simulink model "test_direct"  (R2024a)
settings: Solver=VariableStepAuto  StartTime=0.0  StopTime=40  RelTol=1e-3
libraries: neural x733, simulink x4
(part 24 of 35)

== system test_direct/Function Fitting Neural Network4/Layer 4/Delays 1 ==
  "p{4}" : Inport  PortDimensions=20
      mask Display: e = 0.06;c1 = [120 230 180]/255;c2 = ([120 230 180]+0)/(256+128);c3 = ([120 230 180]+128)/(256+128);patch([0 1 1 0],[0 0 1 1],c1);patch([0 1 1 1-e 1-e 0+e],[0 0 1 1-e 0+e 0+e],c2);patch([0 0 1 1-e 0+e 0+e],[0 1 1 1-e 1-e 0+e],c3);plot([0 1 1 0 0],[0 0 1 1 0]);
  mux : Mux  Inputs=1
      mask Display: e = 0.06;c1 = [120 150 230]/255;c2 = ([120 150 230]+0)/383;c3 = ([120 150 230]+128)/383;patch([0 1 1 0],[0 0 1 1],c1);patch([0 1 1 1-e 1-e 0+e],[0 0 1 1-e 0+e 0+e],c2);patch([0 0 1 1-e 0+e 0+e],[0 1 1 1-e 1-e 0+e],c3);plot([0 1 1 0 0],[0 0 1 1 0]);disp('Mux')
  "pd{4,3}" : Outport
      mask Display: e = 0.06;c1 = [120 230 180]/255;c2 = ([120 230 180]+0)/(256+128);c3 = ([120 230 180]+128)/(256+128);patch([0 1 1 0],[0 0 1 1],c1);patch([0 1 1 1-e 1-e 0+e],[0 0 1 1-e 0+e 0+e],c2);patch([0 0 1 1-e 0+e 0+e],[0 1 1 1-e 1-e 0+e],c3);plot([0 1 1 0 0],[0 0 1 1 0]);
  wires:
  "p{4}"/1 -> mux/1
  mux/1 -> "pd{4,3}"/1

== system test_direct/Function Fitting Neural Network4/Layer 4/LW{4,3} ==
  "ad{4,3}" : Inport  PortDimensions=20
      mask Display: e = 0.06;c1 = [120 230 180]/255;c2 = ([120 230 180]+0)/(256+128);c3 = ([120 230 180]+128)/(256+128);patch([0 1 1 0],[0 0 1 1],c1);patch([0 1 1 1-e 1-e 0+e],[0 0 1 1-e 0+e 0+e],c2);patch([0 0 1 1-e 0+e 0+e],[0 1 1 1-e 1-e 0+e],c3);plot([0 1 1 0 0],[0 0 1 1 0]);
  "IW{4,3}(1,:)'" : Constant  Value=[-0.0182808475685428926948983274769489071331918239593505859375;0.0804580234912133374081122383358888328075408935546875;-0.2073100011052473601314005691165220923721790313720703125;-0.56877624107405078124344299794756807386875152587890625;-0.37106551095573958587436891320976428687572479248046875;0.2453467469113256027579694773521623574197292327880859375;-0.1097157740776300016705135931260883808135986328125;0.293030747380307599048165911881369538605213165283203125;0.4286556952932023545344009107793681323528289794921875;-0.2927619933728118351012881248607300221920013427734375;-0.330831802187190826547436017790460027754306793212890625;-0.01300416253790542993329371057598109473474323749542236328125;-0.220024597925029985479028482586727477610111236572265625;0.28856741284184350693209353266865946352481842041015625;0.1738140495019694087286410422166227363049983978271484375;0.57653717402246307255353485743398778140544891357421875;-0.08144393527626341000580367790462332777678966522216796875;0.62386015914583803354531710283481515944004058837890625;0.23299635893419512466806509110028855502605438232421875;0.462827846568813539018805158775649033486843109130859375]
      mask Display: e = 0.06;c1 = [120 150 230]/255;c2 = ([120 150 230]+0)/383;c3 = ([120 150 230]+128)/383;patch([0 1 1 0],[0 0 1 1],c1);patch([0 1 1 1-e 1-e 0+e],[0 0 1 1-e 0+e 0+e],c2);patch([0 0 1 1-e 0+e 0+e],[0 1 1 1-e 1-e 0+e],c3);plot([0 1 1 0 0],[0 0 1 1 0]);disp('weights');
  "IW{4,3}(10,:)'" : Constant  Value=[-0.5867021051616487792301768422476015985012054443359375;-0.40646884911088843050919194865855388343334197998046875;0.1384930279966194444085658687981776893138885498046875;0.60431005202610743598512499374919570982456207275390625;0.231549088394502333709823460594634525477886199951171875;-0.278578383513912342106522146423230879008769989013671875;-0.2401723445859841599148154500653618015348911285400390625;-0.278682695857914330961335735992179252207279205322265625;0.389949189397055973049788235584856010973453521728515625;-0.378849241372464284882681795352254994213581085205078125;-0.50446895043893802412782179089845158159732818603515625;-0.04123499520558514264134686300167231820523738861083984375;-0.412512646032147267671774670816375873982906341552734375;0.0298074784018579376498880861845464096404612064361572265625;-0.6030020171920196236925448829424567520618438720703125;-0.0918971849790183037409718735943897627294063568115234375;-0.1048877360115925416739202091775950975716114044189453125;0.426138672134914464617594376250053755939006805419921875;-0.028373006982034938705528048785708961077034473419189453125;-0.10103546567123274091404283581141498871147632598876953125]
      mask Display: e = 0.06;c1 = [120 150 230]/255;c2 = ([120 150 230]+0)/383;c3 = ([120 150 230]+128)/383;patch([0 1 1 0],[0 0 1 1],c1);patch([0 1 1 1-e 1-e 0+e],[0 0 1 1-e 0+e 0+e],c2);patch([0 0 1 1-e 0+e 0+e],[0 1 1 1-e 1-e 0+e],c3);plot([0 1 1 0 0],[0 0 1 1 0]);disp('weights');
  "IW{4,3}(2,:)'" : Constant  Value=[0.04766233737430193573292314113132306374609470367431640625;0.472662950403235637697463289441657252609729766845703125;0.393481975518174265094017982846708036959171295166015625;-0.4054200644776970730021048439084552228450775146484375;0.64596436275341506672020841506309807300567626953125;0.34833116550052078963517487864010035991668701171875;0.0158927016381227755037475191102203098125755786895751953125;0.1432191124397620696218069724636734463274478912353515625;-0.1525863659129366445288411568981246091425418853759765625;-0.08213514792309771495038006605682312510907649993896484375;-0.05352653335257491484799885483880643732845783233642578125;-0.2237879229032577743652154822484590113162994384765625;-0.251639048104404128292088671514648012816905975341796875;0.374060271638200159127762844946119002997875213623046875;-0.13843849114586415094407811920973472297191619873046875;-0.00157935386633405584581868463800446988898329436779022216796875;0.08123459901137251859548626953255734406411647796630859375;-0.60194027599860344679427726077847182750701904296875;-0.2419573839009540316968838169486843980848789215087890625;0.4202479369474840797948900217306800186634063720703125]
      mask Display: e = 0.06;c1 = [120 150 230]/255;c2 = ([120 150 230]+0)/383;c3 = ([120 150 230]+128)/383;patch([0 1 1 0],[0 0 1 1],c1);patch([0 1 1 1-e 1-e 0+e],[0 0 1 1-e 0+e 0+e],c2);patch([0 0 1 1-e 0+e 0+e],[0 1 1 1-e 1-e 0+e],c3);plot([0 1 1 0 0],[0 0 1 1 0]);disp('weights');
  "IW{4,3}(3,:)'" : Constant  Value=[0.64653136532270083502993429647176526486873626708984375;-0.17598643231509558670921933298814110457897186279296875;-0.3306166204372065209327047341503202915191650390625;0.5500686330664434908754856223822571337223052978515625;-0.258915156366846421764904562223819084465503692626953125;-0.2135157354375183669237259209694457240402698516845703125;0.0280209258454371910873614837100831209681928157806396484375;0.023128965179387513118047792204379220493137836456298828125;0.300633725443321286885378640363342128694057464599609375;0.34519443371440450274434397215372882783412933349609375;-0.307061664525679400838953370111994445323944091796875;0.0201426192713053155147751027698177495039999485015869140625;0.1928095450190112358779259693619678728282451629638671875;-0.2828180192111175994540417377720586955547332763671875;0.67880942307011460368215693961246870458126068115234375;-0.18199528762274497228901282142032869160175323486328125;0.15160314165136490327512319709057919681072235107421875;0.48788420536031595897696888641803525388240814208984375;0.1995805530883998091251640971677261404693126678466796875;-0.39812724429761658928583756278385408222675323486328125]
      mask Display: e = 0.06;c1 = [120 150 230]/255;c2 = ([120 150 230]+0)/383;c3 = ([120 150 230]+128)/383;patch([0 1 1 0],[0 0 1 1],c1);patch([0 1 1 1-e 1-e 0+e],[0 0 1 1-e 0+e 0+e],c2);patch([0 0 1 1-e 0+e 0+e],[0 1 1 1-e 1-e 0+e],c3);plot([0 1 1 0 0],[0 0 1 1 0]);disp('weights');
  "IW{4,3}(4,:)'" : Constant  Value=[0.46897639649297795383375841993256472051143646240234375;0.1353316784521863269663555229271878488361835479736328125;-0.4090318643737698156570559149258770048618316650390625;-0.10034667176648993935916820419151918031275272369384765625;0.15356197843960306403943150144186802208423614501953125;-0.74982192036332262485842647947720251977443695068359375;0.736163475218127860699723896686919033527374267578125;-0.388099606476475178507001828620559535920619964599609375;0.1284378189965413030737551025595166720449924468994140625;-0.35342224141770184342448146708193235099315643310546875;0.33768468281888275317470515801687724888324737548828125;-0.33768459631601943637946305898367427289485931396484375;0.339246448835974323543496211641468107700347900390625;-0.182148817954333519519849460266414098441600799560546875;-0.45675022943742826786461819210671819746494293212890625;-0.1308331396638943433519131076536723412573337554931640625;0.007235920518857773438281544287065116805024445056915283203125;-0.2181989741993194120706078820148832164704799652099609375;0.697710740419517083665823520277626812458038330078125;0.03270757109621826030920743733076960779726505279541015625]
      mask Display: e = 0.06;c1 = [120 150 230]/255;c2 = ([120 150 230]+0)/383;c3 = ([120 150 230]+128)/383;patch([0 1 1 0],[0 0 1 1],c1);patch([0 1 1 1-e 1-e 0+e],[0 0 1 1-e 0+e 0+e],c2);patch([0 0 1 1-e 0+e 0+e],[0 1 1 1-e 1-e 0+e],c3);plot([0 1 1 0 0],[0 0 1 1 0]);disp('weights');
  "IW{4,3}(5,:)'" : Constant  Value=[0.254012415241254452258345963855390436947345733642578125;-0.278201611801674075774570837893406860530376434326171875;-0.130987915740999272262712338488199748098850250244140625;0.65659498971948615508864577350323088467121124267578125;-0.37010577209780526342086659496999345719814300537109375;-0.364239904557088711722911966717219911515712738037109375;-0.346218175332081823381003005124512128531932830810546875;-0.131514115645591733727570726841804571449756622314453125;-0.16293218459890457250338613448548130691051483154296875;-0.07690950801719813323398255988649907521903514862060546875;-0.04995568746558680384151074349574628286063671112060546875;-0.297894174787131815751450858442694880068302154541015625;-0.208190351516119920294300982277491129934787750244140625;-0.13629072817438714348980965951341204345226287841796875;-0.384110184134717147497184441817807964980602264404296875;-0.43900730118536801516171408366062678396701812744140625;0.0692901289663383213035530161505448631942272186279296875;0.27697027123827278050072209225618280470371246337890625;0.0208057391676239288036409647020263946615159511566162109375;0.6856311827603163155941956574679352343082427978515625]
      mask Display: e = 0.06;c1 = [120 150 230]/255;c2 = ([120 150 230]+0)/383;c3 = ([120 150 230]+128)/383;patch([0 1 1 0],[0 0 1 1],c1);patch([0 1 1 1-e 1-e 0+e],[0 0 1 1-e 0+e 0+e],c2);patch([0 0 1 1-e 0+e 0+e],[0 1 1 1-e 1-e 0+e],c3);plot([0 1 1 0 0],[0 0 1 1 0]);disp('weights');
  "IW{4,3}(6,:)'" : Constant  Value=[0.06383515321962386634968567022951901890337467193603515625;-0.348969499010585881837442912001279182732105255126953125;-0.67269644646642923202506381130660884082317352294921875;0.44685601061213520157622269834973849356174468994140625;-0.358281232233862712011074336260207928717136383056640625;0.07916658582745154937310161358254845254123210906982421875;0.30505773608176711686468252082704566419124603271484375;0.617951579143801499327537385397590696811676025390625;-0.25294218554518221875326844383380375802516937255859375;-0.3977997598759459574324637287645600736141204833984375;0.058739564042513479902307693691909662447869777679443359375;0.1494537664697459522500366801978088915348052978515625;0.60851330942889114705707243047072552144527435302734375;-0.055559362022579848738867980273425928317010402679443359375;-0.62443423379172180442964190660859458148479461669921875;-0.2268644620133335454426060096011497080326080322265625;-0.57816378248105604331641416138154454529285430908203125;0.39207408987547409662255404327879659831523895263671875;-0.074342103653326108148036155398585833609104156494140625;0.285697237530900871593786405355785973370075225830078125]
      mask Display: e = 0.06;c1 = [120 150 230]/255;c2 = ([120 150 230]+0)/383;c3 = ([120 150 230]+128)/383;patch([0 1 1 0],[0 0 1 1],c1);patch([0 1 1 1-e 1-e 0+e],[0 0 1 1-e 0+e 0+e],c2);patch([0 0 1 1-e 0+e 0+e],[0 1 1 1-e 1-e 0+e],c3);plot([0 1 1 0 0],[0 0 1 1 0]);disp('weights');
  "IW{4,3}(7,:)'" : Constant  Value=[0.1735578250848583692356186247707228176295757293701171875;-0.1443796965013408317712872985794092528522014617919921875;-0.00192713703805364963174417969327123500988818705081939697265625;-0.050944766962450170610932076442622928880155086517333984375;-0.56313960947635821607804018640308640897274017333984375;0.406795735506861155794666728979791514575481414794921875;-0.43477191912486556901740186731331050395965576171875;-0.0183635163924778209432187026095562032423913478851318359375;-0.16499808196158738393677367639611475169658660888671875;0.1554097258561016603461979457279085181653499603271484375;-0.45712271023931894120551078231073915958404541015625;-0.31639810290967407269135946989990770816802978515625;0.283675985048455980841453083485248498618602752685546875;-0.434852696669257132722208325503743253648281097412109375;0.184268928265691245282908994340687058866024017333984375;0.487799544058790834899497212973074056208133697509765625;-0.1646897501250245976489594568192842416465282440185546875;0.55969685707381255923564822296611964702606201171875;-0.40425367209081686237226449520676396787166595458984375;0.259423740372571154377823177128448151051998138427734375]
      mask Display: e = 0.06;c1 = [120 150 230]/255;c2 = ([120 150 230]+0)/383;c3 = ([120 150 230]+128)/383;patch([0 1 1 0],[0 0 1 1],c1);patch([0 1 1 1-e 1-e 0+e],[0 0 1 1-e 0+e 0+e],c2);patch([0 0 1 1-e 0+e 0+e],[0 1 1 1-e 1-e 0+e],c3);plot([0 1 1 0 0],[0 0 1 1 0]);disp('weights');
  "IW{4,3}(8,:)'" : Constant  Value=[-0.044604630833756091223829542968815076164901256561279296875;0.1653273492054885551727494430451770313084125518798828125;0.35228947713259184393308487415197305381298065185546875;0.388185803066177392839364301835303194820880889892578125;0.59881679713870406001063884104951284825801849365234375;-0.07736001152979880834958947843915666453540325164794921875;-0.5271011175306501428394767572171986103057861328125;-0.09774032952107626626148118020864785648882389068603515625;0.18675638954029449845251065198681317269802093505859375;-0.478571423377917526398306335977395065128803253173828125;0.34027059434836159912407538286061026155948638916015625;0.057705036219698628563445907957429881207644939422607421875;-0.214782881199087782864154405615408904850482940673828125;-0.26706306507587018739258155619609169661998748779296875;-0.54002602442711433727851044750423170626163482666015625;0.58528571806826767964793134524370543658733367919921875;0.030194751746646243673044551769635290838778018951416015625;-0.4346282259921803170499288171413354575634002685546875;0.40357189348227062719587365791085176169872283935546875;0.193904249336287748395335484019597060978412628173828125]
      mask Display: e = 0.06;c1 = [120 150 230]/255;c2 = ([120 150 230]+0)/383;c3 = ([120 150 230]+128)/383;patch([0 1 1 0],[0 0 1 1],c1);patch([0 1 1 1-e 1-e 0+e],[0 0 1 1-e 0+e 0+e],c2);patch([0 0 1 1-e 0+e 0+e],[0 1 1 1-e 1-e 0+e],c3);plot([0 1 1 0 0],[0 0 1 1 0]);disp('weights');
  "IW{4,3}(9,:)'" : Constant  Value=[-0.262696724536377546055376797085045836865901947021484375;-0.495272708083491608466175648572971113026142120361328125;-0.3543852059837149237608855401049368083477020263671875;-0.221393523730061769771992885580402798950672149658203125;-0.038436478394411034698041618185015977360308170318603515625;-0.318611608590077199920642669894732534885406494140625;-0.07339652443837078876764934420862118713557720184326171875;1.061095964250348355761843777145259082317352294921875;-0.4127361165109009188967092995881102979183197021484375;-0.025399426654827285398940972527270787395536899566650390625;-0.5236953508005728341601070496835745871067047119140625;-0.335822568857687187016125562877277843654155731201171875;0.350185935701288586496815469217835925519466400146484375;-0.195141267318745648129407754822750575840473175048828125;0.9131446131154741241431338494294323027133941650390625;-0.4326775227891754838083215872757136821746826171875;-0.63697775880777218748818313542869873344898223876953125;0.55100216042612715217074992324342019855976104736328125;-0.09919080628567943092033232233006856404244899749755859375;0.134968530413840992476792735033086501061916351318359375]
      mask Display: e = 0.06;c1 = [120 150 230]/255;c2 = ([120 150 230]+0)/383;c3 = ([120 150 230]+128)/383;patch([0 1 1 0],[0 0 1 1],c1);patch([0 1 1 1-e 1-e 0+e],[0 0 1 1-e 0+e 0+e],c2);patch([0 0 1 1-e 0+e 0+e],[0 1 1 1-e 1-e 0+e],c3);plot([0 1 1 0 0],[0 0 1 1 0]);disp('weights');
  Mux : Mux  Inputs=10
      mask Display: e = 0.06;c1 = [120 150 230]/255;c2 = ([120 150 230]+0)/383;c3 = ([120 150 230]+128)/383;patch([0 1 1 0],[0 0 1 1],c1);patch([0 1 1 1-e 1-e 0+e],[0 0 1 1-e 0+e 0+e],c2);patch([0 0 1 1-e 0+e 0+e],[0 1 1 1-e 1-e 0+e],c3);plot([0 1 1 0 0],[0 0 1 1 0]);disp('Mux');
  dotprod{1..10} (10 alike) : neural/Weight Functions/dotprod
  "lz{4,3}" : Outport
      mask Display: e = 0.06;c1 = [120 230 180]/255;c2 = ([120 230 180]+0)/(256+128);c3 = ([120 230 180]+128)/(256+128);patch([0 1 1 0],[0 0 1 1],c1);patch([0 1 1 1-e 1-e 0+e],[0 0 1 1-e 0+e 0+e],c2);patch([0 0 1 1-e 0+e 0+e],[0 1 1 1-e 1-e 0+e],c3);plot([0 1 1 0 0],[0 0 1 1 0]);
  wires:
  "IW{4,3}(1,:)'"/1 -> dotprod1/1
  "ad{4,3}"/1 -> dotprod1/2, dotprod2/2, dotprod3/2, dotprod4/2, dotprod5/2, dotprod6/2, dotprod7/2, dotprod8/2, dotprod9/2, dotprod10/2
  dotprod1/1 -> Mux/1
  "IW{4,3}(2,:)'"/1 -> dotprod2/1
  dotprod2/1 -> Mux/2
  "IW{4,3}(3,:)'"/1 -> dotprod3/1
  dotprod3/1 -> Mux/3
  "IW{4,3}(4,:)'"/1 -> dotprod4/1
  dotprod4/1 -> Mux/4
  "IW{4,3}(5,:)'"/1 -> dotprod5/1
  dotprod5/1 -> Mux/5
  "IW{4,3}(6,:)'"/1 -> dotprod6/1
  dotprod6/1 -> Mux/6
  "IW{4,3}(7,:)'"/1 -> dotprod7/1
  dotprod7/1 -> Mux/7
  "IW{4,3}(8,:)'"/1 -> dotprod8/1
  dotprod8/1 -> Mux/8
  "IW{4,3}(9,:)'"/1 -> dotprod9/1
  dotprod9/1 -> Mux/9
  "IW{4,3}(10,:)'"/1 -> dotprod10/1
  dotprod10/1 -> Mux/10
  Mux/1 -> "lz{4,3}"/1

== system test_direct/Function Fitting Neural Network4/Layer 5/Delays 1 ==
  "p{5}" : Inport  PortDimensions=10
      mask Display: e = 0.06;c1 = [120 230 180]/255;c2 = ([120 230 180]+0)/(256+128);c3 = ([120 230 180]+128)/(256+128);patch([0 1 1 0],[0 0 1 1],c1);patch([0 1 1 1-e 1-e 0+e],[0 0 1 1-e 0+e 0+e],c2);patch([0 0 1 1-e 0+e 0+e],[0 1 1 1-e 1-e 0+e],c3);plot([0 1 1 0 0],[0 0 1 1 0]);
  mux : Mux  Inputs=1
      mask Display: e = 0.06;c1 = [120 150 230]/255;c2 = ([120 150 230]+0)/383;c3 = ([120 150 230]+128)/383;patch([0 1 1 0],[0 0 1 1],c1);patch([0 1 1 1-e 1-e 0+e],[0 0 1 1-e 0+e 0+e],c2);patch([0 0 1 1-e 0+e 0+e],[0 1 1 1-e 1-e 0+e],c3);plot([0 1 1 0 0],[0 0 1 1 0]);disp('Mux')
  "pd{5,4}" : Outport
      mask Display: e = 0.06;c1 = [120 230 180]/255;c2 = ([120 230 180]+0)/(256+128);c3 = ([120 230 180]+128)/(256+128);patch([0 1 1 0],[0 0 1 1],c1);patch([0 1 1 1-e 1-e 0+e],[0 0 1 1-e 0+e 0+e],c2);patch([0 0 1 1-e 0+e 0+e],[0 1 1 1-e 1-e 0+e],c3);plot([0 1 1 0 0],[0 0 1 1 0]);
  wires:
  "p{5}"/1 -> mux/1
  mux/1 -> "pd{5,4}"/1

== system test_direct/Function Fitting Neural Network4/Layer 5/LW{5,4} ==
  "ad{5,4}" : Inport  PortDimensions=10
      mask Display: e = 0.06;c1 = [120 230 180]/255;c2 = ([120 230 180]+0)/(256+128);c3 = ([120 230 180]+128)/(256+128);patch([0 1 1 0],[0 0 1 1],c1);patch([0 1 1 1-e 1-e 0+e],[0 0 1 1-e 0+e 0+e],c2);patch([0 0 1 1-e 0+e 0+e],[0 1 1 1-e 1-e 0+e],c3);plot([0 1 1 0 0],[0 0 1 1 0]);
  "IW{5,4}(1,:)'" : Constant  Value=[-0.609586613853234648985335297766141593456268310546875;-0.991992343621268535258650445030070841312408447265625;0.55645920623334166332796257847803644835948944091796875;-0.2756548382209949021870443175430409610271453857421875;0.79182679604217509616859160814783535897731781005859375;0.5409353217326822171884259660146199166774749755859375;0.8560146531317720519638214682345278561115264892578125;0.369094621261524424848943226606934331357479095458984375;1.144450010398711636838697813800536096096038818359375;0.82688754328264491011424297539633698761463165283203125]
      mask Display: e = 0.06;c1 = [120 150 230]/255;c2 = ([120 150 230]+0)/383;c3 = ([120 150 230]+128)/383;patch([0 1 1 0],[0 0 1 1],c1);patch([0 1 1 1-e 1-e 0+e],[0 0 1 1-e 0+e 0+e],c2);patch([0 0 1 1-e 0+e 0+e],[0 1 1 1-e 1-e 0+e],c3);plot([0 1 1 0 0],[0 0 1 1 0]);disp('weights');
  "IW{5,4}(2,:)'" : Constant  Value=[-0.2491134788551136736156621509508113376796245574951171875;-0.348638402621329834829566607368178665637969970703125;-0.58928454736647262190984974949969910085201263427734375;1.1057017527083596863946013399981893599033355712890625;0.69839147102565746205726782136480323970317840576171875;-0.78717405206411239504404875333420932292938232421875;0.1763952297557981607756261155373067595064640045166015625;-0.0641150518456101436992611297682742588222026824951171875;-0.9062580556750947646804661417263559997081756591796875;-1.0565207862803387417471867593121714890003204345703125]
      mask Display: e = 0.06;c1 = [120 150 230]/255;c2 = ([120 150 230]+0)/383;c3 = ([120 150 230]+128)/383;patch([0 1 1 0],[0 0 1 1],c1);patch([0 1 1 1-e 1-e 0+e],[0 0 1 1-e 0+e 0+e],c2);patch([0 0 1 1-e 0+e 0+e],[0 1 1 1-e 1-e 0+e],c3);plot([0 1 1 0 0],[0 0 1 1 0]);disp('weights');
  Mux : Mux  Inputs=2
      mask Display: e = 0.06;c1 = [120 150 230]/255;c2 = ([120 150 230]+0)/383;c3 = ([120 150 230]+128)/383;patch([0 1 1 0],[0 0 1 1],c1);patch([0 1 1 1-e 1-e 0+e],[0 0 1 1-e 0+e 0+e],c2);patch([0 0 1 1-e 0+e 0+e],[0 1 1 1-e 1-e 0+e],c3);plot([0 1 1 0 0],[0 0 1 1 0]);disp('Mux');
  dotprod1 : neural/Weight Functions/dotprod
  dotprod2 : neural/Weight Functions/dotprod
  "lz{5,4}" : Outport
      mask Display: e = 0.06;c1 = [120 230 180]/255;c2 = ([120 230 180]+0)/(256+128);c3 = ([120 230 180]+128)/(256+128);patch([0 1 1 0],[0 0 1 1],c1);patch([0 1 1 1-e 1-e 0+e],[0 0 1 1-e 0+e 0+e],c2);patch([0 0 1 1-e 0+e 0+e],[0 1 1 1-e 1-e 0+e],c3);plot([0 1 1 0 0],[0 0 1 1 0]);
  wires:
  "IW{5,4}(1,:)'"/1 -> dotprod1/1
  "ad{5,4}"/1 -> dotprod1/2, dotprod2/2
  dotprod1/1 -> Mux/1
  "IW{5,4}(2,:)'"/1 -> dotprod2/1
  dotprod2/1 -> Mux/2
  Mux/1 -> "lz{5,4}"/1

== system test_direct/Function Fitting Neural Network5/Layer 1/Delays 1 ==
  "p{1}" : Inport  PortDimensions=8
      mask Display: e = 0.06;c1 = [120 230 180]/255;c2 = ([120 230 180]+0)/(256+128);c3 = ([120 230 180]+128)/(256+128);patch([0 1 1 0],[0 0 1 1],c1);patch([0 1 1 1-e 1-e 0+e],[0 0 1 1-e 0+e 0+e],c2);patch([0 0 1 1-e 0+e 0+e],[0 1 1 1-e 1-e 0+e],c3);plot([0 1 1 0 0],[0 0 1 1 0]);
  mux : Mux  Inputs=1
      mask Display: e = 0.06;c1 = [120 150 230]/255;c2 = ([120 150 230]+0)/383;c3 = ([120 150 230]+128)/383;patch([0 1 1 0],[0 0 1 1],c1);patch([0 1 1 1-e 1-e 0+e],[0 0 1 1-e 0+e 0+e],c2);patch([0 0 1 1-e 0+e 0+e],[0 1 1 1-e 1-e 0+e],c3);plot([0 1 1 0 0],[0 0 1 1 0]);disp('Mux')
  "pd{1,1}" : Outport
      mask Display: e = 0.06;c1 = [120 230 180]/255;c2 = ([120 230 180]+0)/(256+128);c3 = ([120 230 180]+128)/(256+128);patch([0 1 1 0],[0 0 1 1],c1);patch([0 1 1 1-e 1-e 0+e],[0 0 1 1-e 0+e 0+e],c2);patch([0 0 1 1-e 0+e 0+e],[0 1 1 1-e 1-e 0+e],c3);plot([0 1 1 0 0],[0 0 1 1 0]);
  wires:
  "p{1}"/1 -> mux/1
  mux/1 -> "pd{1,1}"/1

== system test_direct/Function Fitting Neural Network5/Layer 1/IW{1,1} ==
  "pd{1,1}" : Inport  PortDimensions=8
      mask Display: e = 0.06;c1 = [120 230 180]/255;c2 = ([120 230 180]+0)/(256+128);c3 = ([120 230 180]+128)/(256+128);patch([0 1 1 0],[0 0 1 1],c1);patch([0 1 1 1-e 1-e 0+e],[0 0 1 1-e 0+e 0+e],c2);patch([0 0 1 1-e 0+e 0+e],[0 1 1 1-e 1-e 0+e],c3);plot([0 1 1 0 0],[0 0 1 1 0]);
  "IW{1,1}(1,:)'" : Constant  Value=[-0.24282240031374058286672834583441726863384246826171875;-0.265937760938790013209853668740834109485149383544921875;0.120517267596000288154556301378761418163776397705078125;-0.1509670298731921878054862418139236979186534881591796875;-0.83895200425768745589039099286310374736785888671875;-0.90347229810113471870636203675530850887298583984375;0.68495171502979490529838813017704524099826812744140625;0.956494783351313326846820928039960563182830810546875]
      mask Display: e = 0.06;c1 = [120 150 230]/255;c2 = ([120 150 230]+0)/383;c3 = ([120 150 230]+128)/383;patch([0 1 1 0],[0 0 1 1],c1);patch([0 1 1 1-e 1-e 0+e],[0 0 1 1-e 0+e 0+e],c2);patch([0 0 1 1-e 0+e 0+e],[0 1 1 1-e 1-e 0+e],c3);plot([0 1 1 0 0],[0 0 1 1 0]);disp('Weights');
  "IW{1,1}(10,:)'" : Constant  Value=[0.02780686991910841232567008773912675678730010986328125;0.0146068261959116096893041003568214364349842071533203125;-0.2385781861446483187449985052808187901973724365234375;0.1297828418770725911191021850754623301327228546142578125;0.5661070405517631964897873331210575997829437255859375;2.4081053896491244614708193694241344928741455078125;-0.6291887482895004435334840309224091470241546630859375;-0.3738127625013678567711394862271845340728759765625]
      mask Display: e = 0.06;c1 = [120 150 230]/255;c2 = ([120 150 230]+0)/383;c3 = ([120 150 230]+128)/383;patch([0 1 1 0],[0 0 1 1],c1);patch([0 1 1 1-e 1-e 0+e],[0 0 1 1-e 0+e 0+e],c2);patch([0 0 1 1-e 0+e 0+e],[0 1 1 1-e 1-e 0+e],c3);plot([0 1 1 0 0],[0 0 1 1 0]);disp('Weights');
  "IW{1,1}(11,:)'" : Constant  Value=[0.0015329316616055177306676693405051992158405482769012451171875;-0.004795595490663421937849175691326308879069983959197998046875;-0.2186967381351949679668678072630427777767181396484375;-0.04411631562895602931551053416114882566034793853759765625;1.0178167415469101531044771036249585449695587158203125;-0.355344103689434753778897402298753149807453155517578125;-0.9652366094281610298111218071426264941692352294921875;1.957180430553698169404697182471863925457000732421875]
      mask Display: e = 0.06;c1 = [120 150 230]/255;c2 = ([120 150 230]+0)/383;c3 = ([120 150 230]+128)/383;patch([0 1 1 0],[0 0 1 1],c1);patch([0 1 1 1-e 1-e 0+e],[0 0 1 1-e 0+e 0+e],c2);patch([0 0 1 1-e 0+e 0+e],[0 1 1 1-e 1-e 0+e],c3);plot([0 1 1 0 0],[0 0 1 1 0]);disp('Weights');
  "IW{1,1}(12,:)'" : Constant  Value=[0.033997681110883908039976830650630290620028972625732421875;0.037387204982984804935153277938297833316028118133544921875;1.2241007003313961742918536401703022420406341552734375;0.989772821617917575309775202185846865177154541015625;1.015743601330306500329925256664864718914031982421875;0.85100263802785980349341343753621913492679595947265625;-1.09811263426762995010221857228316366672515869140625;0.76300254608823314672605420128093101084232330322265625]
      mask Display: e = 0.06;c1 = [120 150 230]/255;c2 = ([120 150 230]+0)/383;c3 = ([120 150 230]+128)/383;patch([0 1 1 0],[0 0 1 1],c1);patch([0 1 1 1-e 1-e 0+e],[0 0 1 1-e 0+e 0+e],c2);patch([0 0 1 1-e 0+e 0+e],[0 1 1 1-e 1-e 0+e],c3);plot([0 1 1 0 0],[0 0 1 1 0]);disp('Weights');
  "IW{1,1}(13,:)'" : Constant  Value=[-0.00584867446382439197527514096464074100367724895477294921875;-0.014180135875496387154459654311722260899841785430908203125;0.048262697432363992067205771263616043142974376678466796875;-0.04770492383946049741449968450979213230311870574951171875;-0.420740831146248550620470041394582949578762054443359375;0.65870243261579342064493403086089529097080230712890625;0.6527847868744454107314822977059520781040191650390625;-0.2595271311505620293047513769124634563922882080078125]
      mask Display: e = 0.06;c1 = [120 150 230]/255;c2 = ([120 150 230]+0)/383;c3 = ([120 150 230]+128)/383;patch([0 1 1 0],[0 0 1 1],c1);patch([0 1 1 1-e 1-e 0+e],[0 0 1 1-e 0+e 0+e],c2);patch([0 0 1 1-e 0+e 0+e],[0 1 1 1-e 1-e 0+e],c3);plot([0 1 1 0 0],[0 0 1 1 0]);disp('Weights');
  "IW{1,1}(14,:)'" : Constant  Value=[0.3832677484937174750001531720045022666454315185546875;0.236375390594321832526958360176649875938892364501953125;-0.307434790104118338405214672093279659748077392578125;-0.75973655151750119074449685285799205303192138671875;0.6249548206558639407148803002201020717620849609375;0.330795354589032253311842168841394595801830291748046875;1.103439605613709684206469319178722798824310302734375;0.51173857903875286101680330830276943743228912353515625]
      mask Display: e = 0.06;c1 = [120 150 230]/255;c2 = ([120 150 230]+0)/383;c3 = ([120 150 230]+128)/383;patch([0 1 1 0],[0 0 1 1],c1);patch([0 1 1 1-e 1-e 0+e],[0 0 1 1-e 0+e 0+e],c2);patch([0 0 1 1-e 0+e 0+e],[0 1 1 1-e 1-e 0+e],c3);plot([0 1 1 0 0],[0 0 1 1 0]);disp('Weights');
  "IW{1,1}(15,:)'" : Constant  Value=[-0.1830343037830250707553858546816627494990825653076171875;-0.11318758575875147165401557458608294837176799774169921875;0.8364186150389627538714876209269277751445770263671875;0.108692940292483275488422123089549131691455841064453125;-0.8925071740038299505926033816649578511714935302734375;0.37947416924861177012218149684485979378223419189453125;-0.64906408913662427817570232946309261023998260498046875;-0.395045848186393377954317429612274281680583953857421875]
      mask Display: e = 0.06;c1 = [120 150 230]/255;c2 = ([120 150 230]+0)/383;c3 = ([120 150 230]+128)/383;patch([0 1 1 0],[0 0 1 1],c1);patch([0 1 1 1-e 1-e 0+e],[0 0 1 1-e 0+e 0+e],c2);patch([0 0 1 1-e 0+e 0+e],[0 1 1 1-e 1-e 0+e],c3);plot([0 1 1 0 0],[0 0 1 1 0]);disp('Weights');
  "IW{1,1}(16,:)'" : Constant  Value=[-0.01364560598087976965586687327913750777952373027801513671875;-0.04442535095315698623341660322694224305450916290283203125;-1.02925763778331447184655189630575478076934814453125;-0.791757846898343498054373412742279469966888427734375;0.404037544222803524096576666124747134745121002197265625;1.1093011870314255506997369593591429293155670166015625;-0.2280039202570558476423911997699178755283355712890625;-0.78285864379998482132094750340911559760570526123046875]
      mask Display: e = 0.06;c1 = [120 150 230]/255;c2 = ([120 150 230]+0)/383;c3 = ([120 150 230]+128)/383;patch([0 1 1 0],[0 0 1 1],c1);patch([0 1 1 1-e 1-e 0+e],[0 0 1 1-e 0+e 0+e],c2);patch([0 0 1 1-e 0+e 0+e],[0 1 1 1-e 1-e 0+e],c3);plot([0 1 1 0 0],[0 0 1 1 0]);disp('Weights');
  "IW{1,1}(17,:)'" : Constant  Value=[-0.2553234117613261133783453260548412799835205078125;-0.1392227370325401503148299298118217848241329193115234375;0.91924864981972020938627565556089393794536590576171875;0.6145246696287907095523905809386633336544036865234375;-0.95063315123071834289447679111617617309093475341796875;0.0742980094308140770476001080169226042926311492919921875;-0.447293047826839984537627969984896481037139892578125;-0.07736378923439117538674025809086742810904979705810546875]
      mask Display: e = 0.06;c1 = [120 150 230]/255;c2 = ([120 150 230]+0)/383;c3 = ([120 150 230]+128)/383;patch([0 1 1 0],[0 0 1 1],c1);patch([0 1 1 1-e 1-e 0+e],[0 0 1 1-e 0+e 0+e],c2);patch([0 0 1 1-e 0+e 0+e],[0 1 1 1-e 1-e 0+e],c3);plot([0 1 1 0 0],[0 0 1 1 0]);disp('Weights');
  "IW{1,1}(18,:)'" : Constant  Value=[-0.42587133665593823739214940360398031771183013916015625;-0.6138615427850846462121126023703254759311676025390625;-0.2327288350323049315182544205526937730610370635986328125;-0.2276120255623092225594206183814094401895999908447265625;-0.506769106523939694142200096393935382366180419921875;0.308581830945979185276684120253776200115680694580078125;-0.6815697384903725009053232497535645961761474609375;-0.1477754211640225079360533300132374279201030731201171875]
      mask Display: e = 0.06;c1 = [120 150 230]/255;c2 = ([120 150 230]+0)/383;c3 = ([120 150 230]+128)/383;patch([0 1 1 0],[0 0 1 1],c1);patch([0 1 1 1-e 1-e 0+e],[0 0 1 1-e 0+e 0+e],c2);patch([0 0 1 1-e 0+e 0+e],[0 1 1 1-e 1-e 0+e],c3);plot([0 1 1 0 0],[0 0 1 1 0]);disp('Weights');
  "IW{1,1}(19,:)'" : Constant  Value=[0.379732293415370403266706489375792443752288818359375;-0.1595555519094243035471691882776212878525257110595703125;0.950318483165697447390130037092603743076324462890625;-0.89054163698607868848711177633958868682384490966796875;-0.77398786886086490266478676858241669833660125732421875;0.355933090379061900510038185529992915689945220947265625;0.41853242967000114926889864364056847989559173583984375;0.72254742801642490857005896032205782830715179443359375]
      mask Display: e = 0.06;c1 = [120 150 230]/255;c2 = ([120 150 230]+0)/383;c3 = ([120 150 230]+128)/383;patch([0 1 1 0],[0 0 1 1],c1);patch([0 1 1 1-e 1-e 0+e],[0 0 1 1-e 0+e 0+e],c2);patch([0 0 1 1-e 0+e 0+e],[0 1 1 1-e 1-e 0+e],c3);plot([0 1 1 0 0],[0 0 1 1 0]);disp('Weights');
  "IW{1,1}(2,:)'" : Constant  Value=[0.503765398757633153792312441510148346424102783203125;0.34728427513297421835858358463156037032604217529296875;-1.096710226166195401020786448498256504535675048828125;0.462784035857158493332264015407417900860309600830078125;-0.89913794079431463845963889980339445173740386962890625;-0.1626930692858376270581999278874718584120273590087890625;0.369386693508937880014997290345490910112857818603515625;1.0995296511180006060470759621239267289638519287109375]
      mask Display: e = 0.06;c1 = [120 150 230]/255;c2 = ([120 150 230]+0)/383;c3 = ([120 150 230]+128)/383;patch([0 1 1 0],[0 0 1 1],c1);patch([0 1 1 1-e 1-e 0+e],[0 0 1 1-e 0+e 0+e],c2);patch([0 0 1 1-e 0+e 0+e],[0 1 1 1-e 1-e 0+e],c3);plot([0 1 1 0 0],[0 0 1 1 0]);disp('Weights');
  "IW{1,1}(20,:)'" : Constant  Value=[-0.463500722353860583613283097292878665030002593994140625;-0.81599737722350607072030470590107142925262451171875;-0.32719783735946383895765166016644798219203948974609375;-0.40053384670856784222081614643684588372707366943359375;0.63899774146409271669000418114592321217060089111328125;-0.64006294689625675697897122518043033778667449951171875;-0.44045233745919254442213741640443913638591766357421875;-0.08168367648872841557672330736750154756009578704833984375]
      mask Display: e = 0.06;c1 = [120 150 230]/255;c2 = ([120 150 230]+0)/383;c3 = ([120 150 230]+128)/383;patch([0 1 1 0],[0 0 1 1],c1);patch([0 1 1 1-e 1-e 0+e],[0 0 1 1-e 0+e 0+e],c2);patch([0 0 1 1-e 0+e 0+e],[0 1 1 1-e 1-e 0+e],c3);plot([0 1 1 0 0],[0 0 1 1 0]);disp('Weights');
  "IW{1,1}(3,:)'" : Constant  Value=[0.0723748364916112496558753264253027737140655517578125;0.06899037104716111701296910041492083109915256500244140625;0.0231040778098698072751115972778279683552682399749755859375;0.01373786016838408723106379483169803279452025890350341796875;-0.36868446239069119219067260928568430244922637939453125;0.7486580629124144348196523424121551215648651123046875;-0.2346237311682986825811525477547547779977321624755859375;-1.0772597850419514120545727564604021608829498291015625]
      mask Display: e = 0.06;c1 = [120 150 230]/255;c2 = ([120 150 230]+0)/383;c3 = ([120 150 230]+128)/383;patch([0 1 1 0],[0 0 1 1],c1);patch([0 1 1 1-e 1-e 0+e],[0 0 1 1-e 0+e 0+e],c2);patch([0 0 1 1-e 0+e 0+e],[0 1 1 1-e 1-e 0+e],c3);plot([0 1 1 0 0],[0 0 1 1 0]);disp('Weights');
  "IW{1,1}(4,:)'" : Constant  Value=[-0.01154571316516157623854876845825856435112655162811279296875;-0.015918434301198040869973482358545879833400249481201171875;-0.33500553416689882180179438364575617015361785888671875;-0.1741814446284809247966762768555781804025173187255859375;1.0290956808094076091464330602320842444896697998046875;-0.25840013824531415931318178991205058991909027099609375;-0.86294512365705833278894942850456573069095611572265625;1.9706795080646621887154879004810936748981475830078125]
      mask Display: e = 0.06;c1 = [120 150 230]/255;c2 = ([120 150 230]+0)/383;c3 = ([120 150 230]+128)/383;patch([0 1 1 0],[0 0 1 1],c1);patch([0 1 1 1-e 1-e 0+e],[0 0 1 1-e 0+e 0+e],c2);patch([0 0 1 1-e 0+e 0+e],[0 1 1 1-e 1-e 0+e],c3);plot([0 1 1 0 0],[0 0 1 1 0]);disp('Weights');
  "IW{1,1}(5,:)'" : Constant  Value=[-0.01049457889926454744189410206445245421491563320159912109375;-0.035729863245095937196449398243203177116811275482177734375;-0.430774484447114358598440730929723940789699554443359375;-0.0402661741306189480127386559615842998027801513671875;-0.176857648442543757827394301784806884825229644775390625;0.092448046676315509539989534459891729056835174560546875;0.155069558594852330291047337595955468714237213134765625;2.11663540805323346916111404425464570522308349609375]
      mask Display: e = 0.06;c1 = [120 150 230]/255;c2 = ([120 150 230]+0)/383;c3 = ([120 150 230]+128)/383;patch([0 1 1 0],[0 0 1 1],c1);patch([0 1 1 1-e 1-e 0+e],[0 0 1 1-e 0+e 0+e],c2);patch([0 0 1 1-e 0+e 0+e],[0 1 1 1-e 1-e 0+e],c3);plot([0 1 1 0 0],[0 0 1 1 0]);disp('Weights');
  "IW{1,1}(6,:)'" : Constant  Value=[-0.051120531659696322179797789431177079677581787109375;-0.1469645095613345830987128692868282087147235870361328125;-0.1943630337617625880586302855590474791824817657470703125;-0.0862961248053733254170793998127919621765613555908203125;0.2213018685352453884807033546167076565325260162353515625;-0.463147109011033009107194402531604282557964324951171875;-0.2054205721774859938477675314061343669891357421875;-1.9274833003906526318615988202509470283985137939453125]
      mask Display: e = 0.06;c1 = [120 150 230]/255;c2 = ([120 150 230]+0)/383;c3 = ([120 150 230]+128)/383;patch([0 1 1 0],[0 0 1 1],c1);patch([0 1 1 1-e 1-e 0+e],[0 0 1 1-e 0+e 0+e],c2);patch([0 0 1 1-e 0+e 0+e],[0 1 1 1-e 1-e 0+e],c3);plot([0 1 1 0 0],[0 0 1 1 0]);disp('Weights');
  "IW{1,1}(7,:)'" : Constant  Value=[-0.00350074955720112469814697675474235438741743564605712890625;-0.01146075157482118016261107840136901359073817729949951171875;-0.154440964692578008854439985952922143042087554931640625;-0.06737032278262101991916921406300389207899570465087890625;-1.3233228734849655783278876697295345366001129150390625;0.91760714123268216635409544323920272290706634521484375;1.3691568614437079620671511293039657175540924072265625;0.373878014397877489471966327982954680919647216796875]
      mask Display: e = 0.06;c1 = [120 150 230]/255;c2 = ([120 150 230]+0)/383;c3 = ([120 150 230]+128)/383;patch([0 1 1 0],[0 0 1 1],c1);patch([0 1 1 1-e 1-e 0+e],[0 0 1 1-e 0+e 0+e],c2);patch([0 0 1 1-e 0+e 0+e],[0 1 1 1-e 1-e 0+e],c3);plot([0 1 1 0 0],[0 0 1 1 0]);disp('Weights');
  "IW{1,1}(8,:)'" : Constant  Value=[-0.0240972952959477883239092221856481046415865421295166015625;-0.0118753658992399833971287392841986729763448238372802734375;-0.73527702222140745025313890437246300280094146728515625;-0.38907272860587360785444843713776208460330963134765625;1.020545316067873020671186168328858911991119384765625;-0.411154739334674612649678238085471093654632568359375;-0.95343221002979039457869703255710192024707794189453125;-0.1531734423163644276399963928270153701305389404296875]
      mask Display: e = 0.06;c1 = [120 150 230]/255;c2 = ([120 150 230]+0)/383;c3 = ([120 150 230]+128)/383;patch([0 1 1 0],[0 0 1 1],c1);patch([0 1 1 1-e 1-e 0+e],[0 0 1 1-e 0+e 0+e],c2);patch([0 0 1 1-e 0+e 0+e],[0 1 1 1-e 1-e 0+e],c3);plot([0 1 1 0 0],[0 0 1 1 0]);disp('Weights');
  "IW{1,1}(9,:)'" : Constant  Value=[0.0047450332710312383144302117443658062256872653961181640625;0.0092865309018203383295553265952548827044665813446044921875;-0.041284326840054286211767475833767093718051910400390625;0.0193521567803049132638903984116041101515293121337890625;-0.234218092953510759191004808599245734512805938720703125;-0.59102796727611262017632043352932669222354888916015625;0.52631472028489623138369779553613625466823577880859375;0.678027589694444099421843930031172931194305419921875]
      mask Display: e = 0.06;c1 = [120 150 230]/255;c2 = ([120 150 230]+0)/383;c3 = ([120 150 230]+128)/383;patch([0 1 1 0],[0 0 1 1],c1);patch([0 1 1 1-e 1-e 0+e],[0 0 1 1-e 0+e 0+e],c2);patch([0 0 1 1-e 0+e 0+e],[0 1 1 1-e 1-e 0+e],c3);plot([0 1 1 0 0],[0 0 1 1 0]);disp('Weights');
  Mux : Mux  Inputs=20
      mask Display: e = 0.06;c1 = [120 150 230]/255;c2 = ([120 150 230]+0)/383;c3 = ([120 150 230]+128)/383;patch([0 1 1 0],[0 0 1 1],c1);patch([0 1 1 1-e 1-e 0+e],[0 0 1 1-e 0+e 0+e],c2);patch([0 0 1 1-e 0+e 0+e],[0 1 1 1-e 1-e 0+e],c3);plot([0 1 1 0 0],[0 0 1 1 0]);disp('Mux');
  dotprod{1..20} (20 alike) : neural/Weight Functions/dotprod
  "iz{1,1}" : Outport
      mask Display: e = 0.06;c1 = [120 230 180]/255;c2 = ([120 230 180]+0)/(256+128);c3 = ([120 230 180]+128)/(256+128);patch([0 1 1 0],[0 0 1 1],c1);patch([0 1 1 1-e 1-e 0+e],[0 0 1 1-e 0+e 0+e],c2);patch([0 0 1 1-e 0+e 0+e],[0 1 1 1-e 1-e 0+e],c3);plot([0 1 1 0 0],[0 0 1 1 0]);
  wires:
  "IW{1,1}(1,:)'"/1 -> dotprod1/1
  "pd{1,1}"/1 -> dotprod1/2, dotprod2/2, dotprod3/2, dotprod4/2, dotprod5/2, dotprod6/2, dotprod7/2, dotprod8/2, dotprod9/2, dotprod10/2, dotprod11/2, dotprod12/2, dotprod13/2, dotprod14/2, dotprod15/2, dotprod16/2, dotprod17/2, dotprod18/2, dotprod19/2, dotprod20/2
  dotprod1/1 -> Mux/1
  "IW{1,1}(2,:)'"/1 -> dotprod2/1
  dotprod2/1 -> Mux/2
  "IW{1,1}(3,:)'"/1 -> dotprod3/1
  dotprod3/1 -> Mux/3
  "IW{1,1}(4,:)'"/1 -> dotprod4/1
  dotprod4/1 -> Mux/4
  "IW{1,1}(5,:)'"/1 -> dotprod5/1
  dotprod5/1 -> Mux/5
  "IW{1,1}(6,:)'"/1 -> dotprod6/1
  dotprod6/1 -> Mux/6
  "IW{1,1}(7,:)'"/1 -> dotprod7/1
  dotprod7/1 -> Mux/7
  "IW{1,1}(8,:)'"/1 -> dotprod8/1
  dotprod8/1 -> Mux/8
  "IW{1,1}(9,:)'"/1 -> dotprod9/1
  dotprod9/1 -> Mux/9
  "IW{1,1}(10,:)'"/1 -> dotprod10/1
  dotprod10/1 -> Mux/10
  "IW{1,1}(11,:)'"/1 -> dotprod11/1
  dotprod11/1 -> Mux/11
  "IW{1,1}(12,:)'"/1 -> dotprod12/1
  dotprod12/1 -> Mux/12
  "IW{1,1}(13,:)'"/1 -> dotprod13/1
  dotprod13/1 -> Mux/13
  "IW{1,1}(14,:)'"/1 -> dotprod14/1
  dotprod14/1 -> Mux/14
  "IW{1,1}(15,:)'"/1 -> dotprod15/1
  dotprod15/1 -> Mux/15
  "IW{1,1}(16,:)'"/1 -> dotprod16/1
  dotprod16/1 -> Mux/16
  "IW{1,1}(17,:)'"/1 -> dotprod17/1
  dotprod17/1 -> Mux/17
  "IW{1,1}(18,:)'"/1 -> dotprod18/1
  dotprod18/1 -> Mux/18
  "IW{1,1}(19,:)'"/1 -> dotprod19/1
  dotprod19/1 -> Mux/19
  "IW{1,1}(20,:)'"/1 -> dotprod20/1
  dotprod20/1 -> Mux/20
  Mux/1 -> "iz{1,1}"/1

== system test_direct/Function Fitting Neural Network5/Layer 2/Delays 1 ==
  "p{2}" : Inport  PortDimensions=20
      mask Display: e = 0.06;c1 = [120 230 180]/255;c2 = ([120 230 180]+0)/(256+128);c3 = ([120 230 180]+128)/(256+128);patch([0 1 1 0],[0 0 1 1],c1);patch([0 1 1 1-e 1-e 0+e],[0 0 1 1-e 0+e 0+e],c2);patch([0 0 1 1-e 0+e 0+e],[0 1 1 1-e 1-e 0+e],c3);plot([0 1 1 0 0],[0 0 1 1 0]);
  mux : Mux  Inputs=1
      mask Display: e = 0.06;c1 = [120 150 230]/255;c2 = ([120 150 230]+0)/383;c3 = ([120 150 230]+128)/383;patch([0 1 1 0],[0 0 1 1],c1);patch([0 1 1 1-e 1-e 0+e],[0 0 1 1-e 0+e 0+e],c2);patch([0 0 1 1-e 0+e 0+e],[0 1 1 1-e 1-e 0+e],c3);plot([0 1 1 0 0],[0 0 1 1 0]);disp('Mux')
  "pd{2,1}" : Outport
      mask Display: e = 0.06;c1 = [120 230 180]/255;c2 = ([120 230 180]+0)/(256+128);c3 = ([120 230 180]+128)/(256+128);patch([0 1 1 0],[0 0 1 1],c1);patch([0 1 1 1-e 1-e 0+e],[0 0 1 1-e 0+e 0+e],c2);patch([0 0 1 1-e 0+e 0+e],[0 1 1 1-e 1-e 0+e],c3);plot([0 1 1 0 0],[0 0 1 1 0]);
  wires:
  "p{2}"/1 -> mux/1
  mux/1 -> "pd{2,1}"/1
